simulink model "trial"  (R2016a)
settings: Solver=VariableStepAuto  StartTime=0.0  StopTime=10.0  RelTol=1e-3
model workspace (MAT data in the model file):
  L = Simulink.Signal
  L.DataType = 'double'
  L.DocUnits = 'm'
  L.Dimensions = 1
  L.DimensionsMode = 'auto'
  L.Complexity = 'real'
  L.SampleTime = -1
  L.SamplingMode = 'auto'
  L.InitialValue = '1.065'
  R = Simulink.Signal
  R.DataType = 'double'
  R.DocUnits = 'm'
  R.Dimensions = 1
  R.DimensionsMode = 'auto'
  R.Complexity = 'real'
  R.SampleTime = -1
  R.SamplingMode = 'auto'
  R.InitialValue = '0.125'
  cb = Simulink.Signal
  cb.DataType = 'double'
  cb.DocUnits = 'm'
  cb.Dimensions = 3
  cb.DimensionsMode = 'auto'
  cb.Complexity = 'real'
  cb.SampleTime = -1
  cb.SamplingMode = 'auto'
  cb.InitialValue = '[0 0 0]'
  cg = Simulink.Signal
  cg.DataType = 'double'
  cg.DocUnits = 'm'
  cg.Dimensions = 3
  cg.DimensionsMode = 'auto'
  cg.Complexity = 'real'
  cg.SampleTime = -1
  cg.SamplingMode = 'Sample based'
  cg.InitialValue = '[0 0 0]'
  m = Simulink.Signal
  m.DataType = 'double'
  m.DocUnits = 'kg'
  m.Dimensions = 1
  m.DimensionsMode = 'auto'
  m.Complexity = 'real'
  m.SampleTime = -1
  m.SamplingMode = 'auto'
  m.InitialValue = '39.00'
  rho = Simulink.Signal
  rho.DataType = 'double'
  rho.DocUnits = 'Kg/m3'
  rho.Dimensions = 1
  rho.DimensionsMode = 'auto'
  rho.Complexity = 'real'
  rho.SampleTime = -1
  rho.SamplingMode = 'auto'
  rho.InitialValue = '1000'
values from neighbouring files (symbols this model uses):
  alpha_AoA = [-12.75 -12.5 -12.25 -12 -11.75 -11.5 -11.25 -11 -10.75 -10.5 -10.25 -10 ... (297 elements, 99x3)]    [alpha_Cd_Cl.mat]
undefined symbols (not defined in the file or in its folder): Thrust_vs_PWM
settings Model: Creator=abhij  LastModifiedBy=abhij

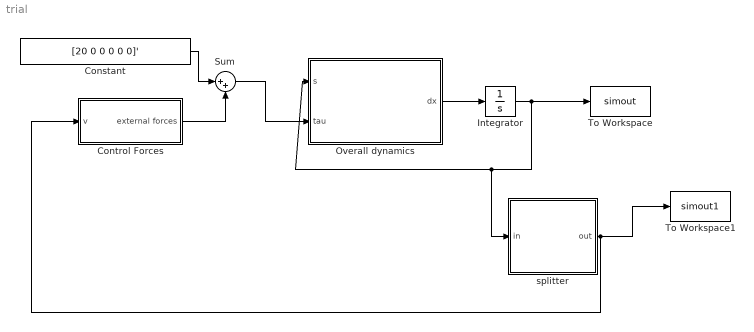
== system trial ==
  Constant : Constant  Value=[20 0 0 0 0 0]'
  Control Forces : Subsystem
  Integrator : Integrator  InitialCondition=zeros(12,1)
  Overall dynamics : MATLAB Function  TreatAsAtomicUnit=on
  Sum : Sum  Inputs=|++
  To Workspace : ToWorkspace  VariableName=simout  SaveFormat=Timeseries  SampleTime=-1
  To Workspace1 : ToWorkspace  VariableName=simout1  SaveFormat=Timeseries  SampleTime=-1
  "splitter " : MATLAB Function  TreatAsAtomicUnit=on
  wires:
  Overall dynamics/1(dx) -> Integrator/1
  Integrator/1 -> To Workspace/1, "splitter "/1(in), Overall dynamics/1(s)
  "splitter "/1(out) -> Control Forces/1(v), To Workspace1/1
  Control Forces/1(external forces) -> Sum/2
  Constant/1 -> Sum/1
  Sum/1 -> Overall dynamics/2(tau)

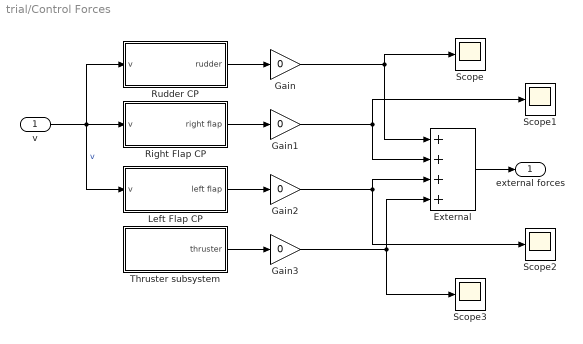
== system trial/Control Forces ==
  v : Inport
  "External " : Sum  Inputs=++++
  Gain{,1..3} (4 alike) : Gain  Gain=0
  Left Flap CP : Subsystem
  Right Flap CP : Subsystem
  Rudder CP : Subsystem
  Scope{,1..3} (4 alike) : Scope
  Thruster subsystem : Subsystem
  external forces : Outport
  wires:
  v/1 -> Rudder CP/1(v), Left Flap CP/1(v), Right Flap CP/1(v)  "v"
  Rudder CP/1("rudder ") -> Gain/1
  "External "/1 -> external forces/1
  Left Flap CP/1(left flap) -> Gain2/1
  Thruster subsystem/1(thruster) -> Gain3/1
  Right Flap CP/1(right flap) -> Gain1/1
  Gain3/1 -> Scope3/1, "External "/4
  Gain2/1 -> Scope2/1, "External "/3
  Gain1/1 -> "External "/2, Scope1/1
  Gain/1 -> "External "/1, Scope/1

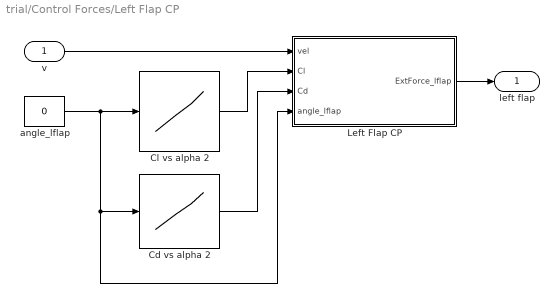
== system trial/Control Forces/Left Flap CP ==
  v : Inport
  Cd vs alpha 2 : Lookup_n-D  NumberOfTableDimensions=1  BreakpointsForDimension1=alpha_AoA(:,1)  Table=alpha_AoA(:,2)  InternalRulePriority=Speed  RndMeth=Simplest  InputSameDT=on
  Cl vs alpha 2 : Lookup_n-D  NumberOfTableDimensions=1  BreakpointsForDimension1=alpha_AoA(:,1)  Table=alpha_AoA(:,3)  InternalRulePriority=Speed  RndMeth=Simplest  InputSameDT=on
  Left Flap CP : MATLAB Function  TreatAsAtomicUnit=on
  angle_lflap : Constant  Value=0
  left flap : Outport
  wires:
  v/1 -> Left Flap CP/1(vel)
  Left Flap CP/1(ExtForce_lflap) -> left flap/1
  angle_lflap/1 -> Left Flap CP/4(angle_lflap), Cd vs alpha 2/1, Cl vs alpha 2/1
  Cl vs alpha 2/1 -> Left Flap CP/2(Cl)
  Cd vs alpha 2/1 -> Left Flap CP/3(Cd)

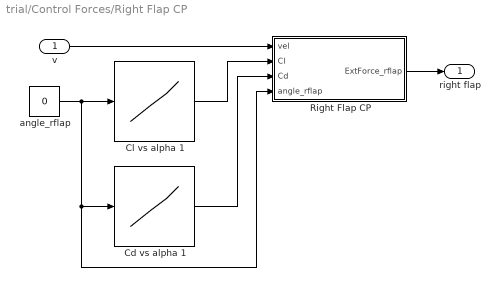
== system trial/Control Forces/Right Flap CP ==
  v : Inport
  Cd vs alpha 1 : Lookup_n-D  NumberOfTableDimensions=1  BreakpointsForDimension1=alpha_AoA(:,1)  Table=alpha_AoA(:,2)  InternalRulePriority=Speed  RndMeth=Simplest  InputSameDT=on
  Cl vs alpha 1 : Lookup_n-D  NumberOfTableDimensions=1  BreakpointsForDimension1=alpha_AoA(:,1)  Table=alpha_AoA(:,3)  InternalRulePriority=Speed  RndMeth=Simplest  InputSameDT=on
  Right Flap CP : MATLAB Function  TreatAsAtomicUnit=on
  angle_rflap : Constant  Value=0
  right flap : Outport
  wires:
  v/1 -> Right Flap CP/1(vel)
  Right Flap CP/1(ExtForce_rflap) -> right flap/1
  Cl vs alpha 1/1 -> Right Flap CP/2(Cl)
  Cd vs alpha 1/1 -> Right Flap CP/3(Cd)
  angle_rflap/1 -> Cl vs alpha 1/1, Cd vs alpha 1/1, Right Flap CP/4(angle_rflap)

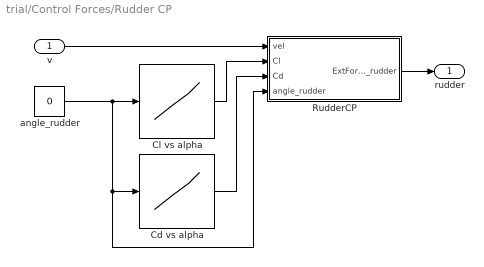
== system trial/Control Forces/Rudder CP ==
  v : Inport
  "Cd vs alpha " : Lookup_n-D  NumberOfTableDimensions=1  BreakpointsForDimension1=alpha_AoA(:,1)  Table=alpha_AoA(:,2)  InternalRulePriority=Speed  RndMeth=Simplest  InputSameDT=on
  "Cl vs alpha " : Lookup_n-D  NumberOfTableDimensions=1  BreakpointsForDimension1=alpha_AoA(:,1)  Table=alpha_AoA(:,3)  InternalRulePriority=Speed  RndMeth=Simplest  InputSameDT=on
  "RudderCP " : MATLAB Function  TreatAsAtomicUnit=on
  angle_rudder : Constant  Value=0
  "rudder " : Outport
  wires:
  v/1 -> "RudderCP "/1(vel)
  "RudderCP "/1(ExtForce_rudder) -> "rudder "/1
  angle_rudder/1 -> "RudderCP "/4(angle_rudder), "Cd vs alpha "/1, "Cl vs alpha "/1
  "Cl vs alpha "/1 -> "RudderCP "/2(Cl)
  "Cd vs alpha "/1 -> "RudderCP "/3(Cd)

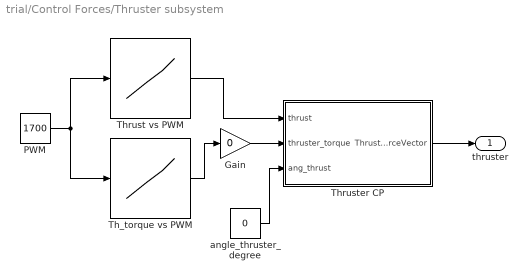
== system trial/Control Forces/Thruster subsystem ==
  Gain : Gain  Gain=0
  PWM : Constant  Value=1700
  Th_torque vs PWM : Lookup_n-D  NumberOfTableDimensions=1  BreakpointsForDimension1=Thrust_vs_PWM(:,1)  BreakpointsForDimension2=Thrust_vs_PWM(:,3)  Table=Thrust_vs_PWM(:,2)  InternalRulePriority=Speed  RndMeth=Simplest  InputSameDT=on
  Thrust vs PWM : Lookup_n-D  NumberOfTableDimensions=1  BreakpointsForDimension1=Thrust_vs_PWM(:,1)  BreakpointsForDimension2=Thrust_vs_PWM(:,3)  Table=Thrust_vs_PWM(:,2)  InternalRulePriority=Speed  RndMeth=Simplest  InputSameDT=on
  Thruster CP : MATLAB Function  TreatAsAtomicUnit=on
  angle_thruster_degree : Constant  Value=0
  thruster : Outport
  wires:
  Thruster CP/1(ThrusterForceVector) -> thruster/1
  PWM/1 -> Thrust vs PWM/1, Th_torque vs PWM/1
  angle_thruster_degree/1 -> Thruster CP/3(ang_thrust)
  Thrust vs PWM/1 -> Thruster CP/1(thrust)
  Gain/1 -> Thruster CP/2(thruster_torque)
  Th_torque vs PWM/1 -> Gain/1

== matlab function trial/splitter  ==
  data: in input; out output
function out = split(in)
out = in(7:12,1);
end

== matlab function trial/Overall dynamics ==
  data: s input; dx output; tau input; cb data_store_memory; cg data_store_memory; m data_store_memory; L data_store_memory; rho data_store_memory; R data_store_memory
function dx = auv_dynamics(s,tau)
% tau = tau';
global cb; %Centre of buyoancy
global cg; %Centre of gravity
global m;%mass of the vehicle
global L;%vehicle length
global rho;%water density
global R;%Radius of the vehicle

x=s(1);
y=s(2);
z=s(3);
pie=s(4);
theta=s(5);
si=s(6);
U=s;

u=s(7);
v=s(8);
w=s(9);
p=s(10);
q=s(11);
r=s(12);

V=[u; v; w; p; q; r];
vel=V;

c_p=cos(pie);
c_t=cos(theta);
c_s=cos(si);
s_p=sin(pie);
s_t=sin(theta);
s_s=sin(si);
t_t=tan(theta);


J1=[c_s*c_t    -s_s*c_p+s_p*s_t*c_s     s_s*s_p+s_t*c_s*c_p;
    s_s*c_t     c_s*c_p+s_p*s_t*s_s    -c_s*s_p+s_t*s_s*c_p;
     -s_t            s_p*c_t                 c_p*c_t       ];
       
J2=[1      s_p*t_t     c_p*t_t;
    0        c_p        -s_p;
    0      s_p/c_t     c_p/c_t ];


J=[J1 zeros(3,3); zeros(3,3) J2];

earth_vel=J*s(7:12);

xdot=earth_vel(1);
ydot=earth_vel(2);
zdot=earth_vel(3);
piedot=earth_vel(4);
thetadot=earth_vel(5);
sidot=earth_vel(6);

%-------------------------------------------------------------------------%
%Sub program for Inertia and added mass matrix  
%
%Values and calculations for Jubilee AUV, 
%developed by Robotics Lab, Department of Engineering Design, IIT Madras
%
%Code modified on 22/07/2011
%By Umesh Neettiyath
%-------------------------------------------------------------------------%
%Use model explorer to modify global variables
%-------------------------------------------------------------------------%

%Centre of gravity
xg=cg(1);yg=cg(2);zg=cg(3);%Centre of gravity

%Inertia values
ixy=0;iyx=ixy;ixz=0;izx=ixz;iyz=0;izy=iyz;
ix=0.34;iy=3.7;iz=3.7;

% Hydrodynamic derivatives
Xudot=-1.170; Xvdot=0; Xwdot=0; Xpdot=0; Xqdot=0; Xrdot=0;
Yudot=0; Yvdot=-34.834; Ywdot=0; Ypdot=0; Yqdot=0; Yrdot=1.042;
Zudot=0; Zvdot=0; Zwdot=-34.834; Zpdot=0; Zqdot=-1.042; Zrdot=0;
Kudot=0; Kvdot=0; Kwdot=0; Kpdot=0; Kqdot=0; Krdot=0;
Mudot=0; Mvdot=0; Mwdot=-1.042; Mpdot=0; Mqdot=-2.659; Mrdot=0; 
Nudot=0; Nvdot=-1.042; Nwdot=0; Npdot=0; Nqdot=0; Nrdot=-2.659;

% Inertia Matrix of Rigid body
M_rb=[m 0 0 0 m*zg -m*yg;...
    0 m 0 -m*zg 0 m*xg;...
    0 0 m m*yg -m*xg 0;...
    0 -m*zg m*yg ix -ixy -ixz;...
    m*zg 0 -m*xg -iyx iy -iyz;...
    -m*yg m*xg 0 -izx -izy iz]; 

% Added Mass matrix
M_a=-[Xudot Xvdot Xwdot Xpdot Xqdot Xrdot;...
    Yudot Yvdot Ywdot Ypdot Yqdot Yrdot;...
    Zudot Zvdot Zwdot Zpdot Zqdot Zrdot;...
    Kudot Kvdot Kwdot Kpdot Kqdot Krdot;...
    Mudot Mvdot Mwdot Mpdot Mqdot Mrdot;...
    Nudot Nvdot Nwdot Npdot Nqdot Nrdot];

% %Total Inertia and mass matrix
%vdot =M\f; %acceleration = inverse(M)*Total force
 
C_rb=[0 0 0 m*(yg*V(5)+zg*V(6)) -m*(xg*V(5)-V(3)) -m*(xg*V(6)+V(2));...
      0 0 0 -m*(yg*V(4)+V(3)) m*(zg*V(6)+xg*V(4)) -m*(yg*V(6)-V(1));...
      0 0 0 -m*(zg*V(4)-V(2)) -m*(zg*V(5)+V(1)) m*(xg*V(4)+yg*V(5));...
      -m*(yg*V(5)+zg*V(6)) m*(yg*V(4)+V(3)) m*(zg*V(4)-V(2)) 0 -iyz*V(5)-ixz*V(4)+iz*V(6) iyz*V(6)+ixy*V(4)-iy*V(5);...
      m*(xg*V(5)-V(3)) -m*(zg*V(6)+xg*V(4)) m*(zg*V(5)+V(1)) iyz*V(5)+ixz*V(4)-iz*V(6) 0 -ixz*V(6)-ixy*V(5)+ix*V(4);...
      m*(xg*V(6)+V(2)) m*(yg*V(6)-V(1)) -m*(xg*V(4)+yg*V(5)) -iyz*V(6)-ixy*V(4)+iy*V(5) ixz*V(6)+ixy*V(5)-ix*V(4) 0];

a1 = Xudot*V(1)+Xvdot*V(2)+Xwdot*V(3)+Xpdot*V(4)+Xqdot*V(5)+Xrdot*V(6);
a2 = Yudot*V(1)+Yvdot*V(2)+Ywdot*V(3)+Ypdot*V(4)+Yqdot*V(5)+Yrdot*V(6);
a3 = Zudot*V(1)+Zvdot*V(2)+Zwdot*V(3)+Zpdot*V(4)+Zqdot*V(5)+Zrdot*V(6);
b1 = Kudot*V(1)+Kvdot*V(2)+Kwdot*V(3)+Kpdot*V(4)+Kqdot*V(5)+Krdot*V(6);
b2 = Mudot*V(1)+Mvdot*V(2)+Mwdot*V(3)+Mpdot*V(4)+Mqdot*V(5)+Mrdot*V(6);
b3 = Nudot*V(1)+Nvdot*V(2)+Nwdot*V(3)+Npdot*V(4)+Nqdot*V(5)+Nrdot*V(6);
  
% Coriolis and Centripetal Forces of Added Mass
c1 = [0 -a3 a2;...
    a3 0 -a1;...
    -a2 a1 0];

c2 = [0 -b3 b2;...
    b3 0 -b1;...
    -b2 b1 0];

C_a=[zeros(3,3) c1;c1 c2];

b=2; %check
xg=cg(1);yg=cg(2);zg=cg(3);%Centre of gravity
xb=cb(1);yb=cb(2);zb=cb(3); % Centre of Buoyancy
W=m*9.81;B=(m+b)*9.81;


%Hydrodynamic derivative details --to be modified for jubilee
Xu=-2.12; Xv=0; Xw=0; Xp=0; Xq=0; Xr=0;
Yu=0; Yv=-62.45; Yw=0; Yp=0; Yq=0; Yr=0.12;
Zu=0; Zv=0; Zw=-0.1749; Zp=0;  Zr=0;Zq=-0.066873;
Ku=0; Kv=0; Kw=0; Kp=0; Kq=0; Kr=0;
Mu=0; Mv=0;  Mp=0;  Mr=0;Mw=0;Mq=0;
Nu=0; Nv=1.2; Nw=0; Np=0; Nq=0; Nr=-31.25;
%jubilee parameters
Xuu=-7.365;Xvv=0;Xww=-0.737;Xpp=0;Xqq=-1.065;Xrr=-1.065;
Yuu=0;Yvv=-112.2;Yww=0;Ypp=0;Yqq=0;Yrr=0.250;
Zuu=0;Zvv=0;Zww=-112.2;Zpp=0;Zqq=-0.250;Zrr=0;
Kuu=0;Kvv=0;Kww=0;Kpp=0;Kqq=0;Krr=0;
Muu=0;Mvv=0;Mww=2.244;Mpp=0;Mqq=-119.5;Mrr=0;
Nuu=0;Nvv=-2.244;Nww=0;Npp=0;Nqq=0;Nrr=-59.75;

% Linear Damping Matrix
Dvl=-[Xu Xv Xw Xp Xq Xr;...
    Yu Yv Yw Yp Yq Yr;...
    Zu Zv Zw Zp Zq Zr;...
    Ku Kv Kw Kp Kq  Kr ;...
    Mu Mv Mw Mp  Mq  Mr ;...
    Nu Nv Nw Np  Nq  Nr ];

% Quadratic Damping Matrix
Dvq = -[Xuu Xvv Xww Xpp Xqq Xrr;...
    Yuu Yvv Yww Ypp Yqq Yrr;...
    Zuu Zvv Zww Zpp Zqq Zrr;...
    Kuu Kvv Kww Kpp Kqq Krr;...
    Muu Mvv Mww Mpp Mqq Mrr;...
    Nuu Nvv Nww Npp Nqq Nrr];

% Restoring efforts
G=[(W-B)*sin(U(5));...
    -(W-B)*cos(U(5))*sin(U(4));...
    -(W-B)*cos(U(5))*cos(U(4));...
    -(yg*W-yb*B)*cos(U(5))*cos(U(4))+(zg*W-zb*B)*cos(U(5))*sin(U(4));...
  (zg*W-zb*B)*sin(U(5))+(xg*W-xb*B)*cos(U(5))*cos(U(4));...
    -(xg*W-xb*B)*cos(U(5))*sin(U(4))-(yg*W-yb*B)*sin(U(5))];


D = Dvl + Dvq;
 
M=M_rb+M_a;
 
C=C_rb+C_a;

accl=M\(tau-(C*vel+D*vel+G));

xddot=accl(1);
yddot=accl(2);
zddot=accl(3);
rollddot=accl(4);
pitchddot=accl(5);
yawddot=accl(6);

dx=[xdot; ydot; zdot; piedot; thetadot; sidot; xddot; yddot; zddot; rollddot; pitchddot; yawddot];

end

== matlab function trial/Control Forces/Rudder CP/RudderCP  ==
  data: vel input; ExtForce_rudder output; Cl input; Cd input; angle_rudder input
function ExtForce_rudder = fcn(vel,Cl,Cd,angle_rudder)

u = vel(1);
v = vel(2);
rho = 1000;

angle_rad = angle_rudder*pi/180;
u0 = u*cos(angle_rad)-v*sin(angle_rad);
v0 = u*sin(angle_rad)+v*cos(angle_rad);

alpha = atan2(v0,u0);
V = u0*cos(alpha)+v0*sin(alpha);

A_rudder = 0.02;
a = 100; b= 200; rx = 135; rz =60; ry = 0;

D = (1/2)*Cl*rho*A_rudder*abs(V)*V;
L = (1/2)*Cd*rho*A_rudder*abs(V)*V;
Fx = (D*cos(angle_rad)-L*sin(angle_rad));
Fy = -(D*sin(angle_rad)+L*cos(angle_rad));
Fz =  0;
Mx = -Fy*(rz+(a/2));
My =  Fx*(rz+(a/2));
Mz =  Fx*(b/2)*sin(angle_rad)+Fy*(rx+(a/2));

ExtForce_rudder = [Fx;Fy;Fz;Mx;My;Mz];

end

== matlab function trial/Control Forces/Right Flap CP/Right Flap CP ==
  data: vel input; ExtForce_rflap output; Cl input; Cd input; angle_rflap input
function ExtForce_rflap = fcn(vel,Cl,Cd,angle_rflap)

u = vel(1);
w = vel(3);
rho = 1000;

angle_rad = angle_rflap*pi/180;
u0 = u*cos(angle_rad)-w*sin(angle_rad);
w0 = u*sin(angle_rad)+w*cos(angle_rad);

alpha = -atan2(w0,u0);
V = u0*cos(alpha)+w0*sin(alpha);

A_rflap = 0.015;
a = 100; b= 150; rx = 90; rz = 30; ry = 88;

D = (1/2)*Cl*rho*A_rflap*V*abs(V);
L = (1/2)*Cd*rho*A_rflap*V*abs(V);
Fx = -(D*cos(angle_rad)+L*sin(angle_rad));
Fy =  0;
Fz =  (D*sin(angle_rad)-L*cos(angle_rad));
Mx =  Fz*(ry+(a/2));
My =  Fx*(rz+(b/2)*sin(angle_rad))+Fz*(rx+(b/2)*cos(angle_rad));
Mz =  Fx*(ry+(a/2));

ExtForce_rflap = [Fx;Fy;Fz;Mx;My;Mz];

end

== matlab function trial/Control Forces/Left Flap CP/Left Flap CP ==
  data: vel input; ExtForce_lflap output; Cl input; Cd input; angle_lflap input
function ExtForce_lflap = fcn(vel,Cl,Cd,angle_lflap)

u = vel(1);
w = vel(3);

angle_rad = angle_lflap*pi/180;
u0 = u*cos(angle_rad)-w*sin(angle_rad);
w0 = u*sin(angle_rad)+w*cos(angle_rad);

rho = 1000;

A_lflap = 0.015;
a = 100; b= 150; rx = 90; rz = 30; ry = 88;

alpha = -atan2(w0,u0);
V = u0*cos(alpha)+w0*sin(alpha);

D = (1/2)*Cl*rho*A_lflap*V*abs(V);
L = (1/2)*Cd*rho*A_lflap*V*abs(V);
Fx = -(D*cos(angle_rad)+L*sin(angle_rad));
Fy =  0;
Fz =  (D*sin(angle_rad)-L*cos(angle_rad));
Mx = -(Fz*(ry+(a/2)));
My =  Fx*(rz+(b/2)*sin(angle_rad))+Fz*(rx+(b/2)*cos(angle_rad));
Mz = -(Fx*(ry+(a/2)));

ExtForce_lflap = [Fx;Fy;Fz;Mx;My;Mz];

end

== matlab function trial/Control Forces/Thruster subsystem/Thruster CP ==
  data: thrust input; thruster_torque input; ThrusterForceVector output; ang_thrust input
function ThrusterForceVector = fcn(thrust,thruster_torque,ang_thrust)

ang_rad_th = ang_thrust*(pi/180);
zth=0;%%%%%%%%%%%%
xth=0.02;
Mth=thruster_torque;

Fx = thrust*cos(ang_rad_th);
Fy = 0;
Fz = thrust*sin(ang_rad_th);
Mx = Mth*cos(ang_rad_th);
My = Fx*zth+Fz*xth;
Mz = Mth*sin(ang_rad_th); 


ThrusterForceVector = [Fx;Fy;Fz;Mx;My;Mz];

end
